simulink model "sldemo_auto_climate_elec"  (Simulink 10.0)
settings: Solver=ode23tb  StartTime=0.0  StopTime=1  RelTol=1e-4  EnableMultiTasking=on
libraries: powerlib x12, simulink x2, simulink_need_slupdate x2
settings Model: FPTRunName=Active  Creator=The MathWorks Inc.  LastModifiedBy=bhisma  ExtModeAutoUpdateStatusClock=off
settings DataIOCC: LimitDataPoints=on  SignalLoggingSaveFormat=ModelDataLogs  SignalLoggingName=sigsOut
settings OptimizationCC: BooleanDataType=off  ExpressionDepthLimit=2147483647  InitFltsAndDblsToZero=on  EfficientMapNaN2IntZero=off
settings DebuggingCC: SaveWithParameterizedLinksMsg=none  SignalResolutionControl=TryResolveAllWithWarning  MultiTaskDSMMsg=warning  MultiTaskCondExecSysMsg=none  FcnCallInpInsideContextMsg=warning  StateNameClashWarn=warning
settings SFSimCC: SimParseCustomCode=off
settings GRTTargetCC: TargetFcnLib=ansi_tfl_tmw.mat  GeneratePreprocessorConditionals=Disable all
settings ConfigComp: CovExternalEMLEnable=off

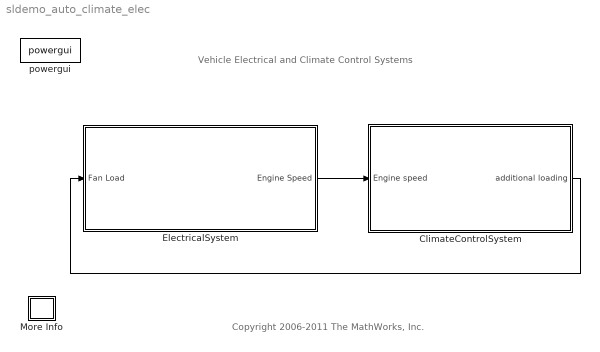
== system sldemo_auto_climate_elec ==
  note: Vehicle Electrical and Climate Control Systems
  note: Copyright 2006-2011 The MathWorks, Inc.
  ClimateControlSystem : Subsystem
  ElectricalSystem : Subsystem
  More Info : Subsystem
      settings: OpenFcn=showdemo(bdroot(gcb))
      mask Display: disp('?')
  powergui : powerlib/powergui  SimulationMode=Continuous  SampleTime=0  frequency=60  Iterations=50  frequencyindice=60  Pbase=100e6  ErrMax=1e-4  UnitsV=kV  UnitsW=MW  buscounter=0  FunctionMessages=off  echomessages=off  EnableUseOfTLC=off  CurrentSourceSwitches=on  DisableSnubberDevices=off  DisableRonSwitches=off  DisableVfSwitches=off  DisplayEquations=off  AutomaticDiscreteSolvers=off  SolverType=Tustin  Interpol=off  ExternalGateDelay=off  methode=off  Ts=0  x0status=blocks  SPID=off  SwTol=0  HookPort=off  NonlinearTolerance=1e-4  nMaxIteration=100  ContinueOnMaxIteration=off  RestoreLinks=no  ResistiveCurrentMeasurement=off  Frange=[0:2:500]  Ylog=off  Xlog=on  ShowGrid=off  save=off  variable=ZData  structure=0  ZoomFFT=on  StartTime=0.0  cycles=1  DisplayStyle=1  fundamental=60  FreqAxis=off  MaxFrequency=1000  frequencyindicesteady=1  RmsSteady=1  display=off
      settings: SourceProductName=Simscape Electrical
  wires:
  ElectricalSystem/1(Engine Speed) -> ClimateControlSystem/1(Engine speed)
  ClimateControlSystem/1(additional loading) -> ElectricalSystem/1(Fan Load)

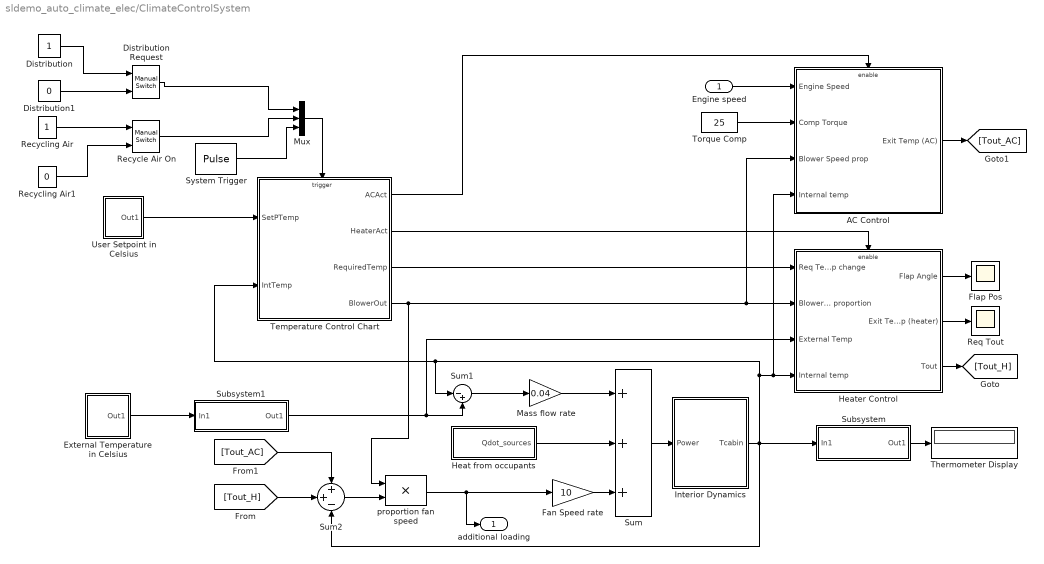
== system sldemo_auto_climate_elec/ClimateControlSystem ==
  Engine speed : Inport
  AC Control : Subsystem  TreatAsAtomicUnit=on
  "Distribution " : Constant
  Distribution Request : simulink/Signal Routing/Manual Switch  sw=0  action=0  varsize=off
      settings: SourceProductName=Simulink  SourceProductBaseCode=SL
  "Distribution1 " : Constant  Value=0
  External Temperature in Celsius : Subsystem  mask(variable){x=18}
      mask prompts: x "Enter the external temperature"
      mask init:
      | set_param('sldemo_auto_climate_elec/ClimateControlSystem/External Temperature in Celsius/External Temp','Value',num2str(x))
      mask Display: disp(x);
  Fan Speed rate : Gain  Gain=10  SaturateOnIntegerOverflow=on  OutDataTypeStr=Inherit: Same as input  ParamDataTypeStr=Inherit: Same as input
  Flap Pos : Scope
  Heat from occupants : Subsystem  mask(Heat from occupants){N=1}
      mask prompts: N "Number of occupants:"
      settings: AttributesFormatString=No. of occupants: %<N>
      mask Display: disp('Heat Sources')
  Heater Control : Subsystem  TreatAsAtomicUnit=on
  Interior Dynamics : Subsystem  mask(Vehicle Cabin Dynamics){}
      mask Display: image(imread([matlabroot,'/toolbox/simulink/simdemos/automotive/html/car_int.jpg']))
  Mass flow rate : Gain  Gain=0.04  SaturateOnIntegerOverflow=on  OutDataTypeStr=Inherit: Same as input  ParamDataTypeStr=Inherit: Same as input
  Mux : Mux  Inputs=3
  Recycle Air On : simulink/Signal Routing/Manual Switch  sw=0  action=0  varsize=off
      settings: SourceProductName=Simulink  SourceProductBaseCode=SL
  Recycling Air : Constant
  Recycling Air1 : Constant  Value=0
  Req Tout : Scope
  Subsystem : Subsystem
      mask Display: disp('Kelvin to Celsius')
  Subsystem1 : Subsystem
      mask Display: disp('Celsius to Kelvin')
  Sum : Sum  Inputs=+++  SaturateOnIntegerOverflow=on  InputSameDT=on  OutDataTypeStr=Inherit: Same as first input
  Sum1 : Sum  Inputs=|-+  SaturateOnIntegerOverflow=on  InputSameDT=on  OutDataTypeStr=Inherit: Same as first input
  Sum2 : Sum  Inputs=++-  SaturateOnIntegerOverflow=on  InputSameDT=on  OutDataTypeStr=Inherit: Same as first input
  System Trigger : DiscretePulseGenerator  PulseType=Time based  Period=1/60  PulseWidth=50
  Temperature Control Chart : Stateflow chart  TreatAsAtomicUnit=on
  Thermometer Display : Display
  Torque Comp : Constant  Value=25
  User Setpoint in Celsius : Subsystem  mask{USet=9}
      mask prompts: USet "Enter the Temperature you require"
      mask init:
      | set_param('sldemo_auto_climate_elec/ClimateControlSystem/User Setpoint in Celsius/User Setpoint','Value',num2str(USet))
      mask Display: disp(num2str(USet))
  proportion fan speed : Product  SaturateOnIntegerOverflow=on  InputSameDT=on  OutDataTypeStr=Inherit: Same as first input
  additional loading : Outport
  wires:
  Distribution Request/1 -> Mux/1
  "Distribution "/1 -> Distribution Request/1
  "Distribution1 "/1 -> Distribution Request/2
  Recycling Air1/1 -> Recycle Air On/2
  User Setpoint in Celsius/1(Out1) -> Temperature Control Chart/1(SetPTemp)
  Recycling Air/1 -> Recycle Air On/1
  Recycle Air On/1 -> Mux/2
  System Trigger/1 -> Mux/3
  Interior Dynamics/1("Tcabin ") -> AC Control/4(Internal temp), Heater Control/4(Internal temp), Temperature Control Chart/2(IntTemp), Sum1/1, Sum2/3, Subsystem/1(In1)
  Subsystem/1(Out1) -> Thermometer Display/1
  Heat from occupants/1(Qdot_sources) -> Sum/2
  External Temperature in Celsius/1(Out1) -> Subsystem1/1(In1)
  Mass flow rate/1 -> Sum/1
  Sum1/1 -> Mass flow rate/1
  Subsystem1/1(Out1) -> Heater Control/3(External Temp), Sum1/2
  Fan Speed rate/1 -> Sum/3
  Sum2/1 -> proportion fan speed/2
  Temperature Control Chart/4(BlowerOut) -> AC Control/3(Blower Speed prop), Heater Control/2(Blower Speed proportion), proportion fan speed/1
  proportion fan speed/1 -> additional loading/1, Fan Speed rate/1
  Temperature Control Chart/2(" HeaterAct") -> Heater Control/Enable
  Heater Control/1(Flap Angle) -> Flap Pos/1
  Heater Control/2(Exit Temp (heater)) -> Req Tout/1
  Heater Control/3(Tout) -> [Tout_H]
  [Tout_H] -> Sum2/2
  Temperature Control Chart/1(" ACAct") -> AC Control/Enable
  [Tout_AC] -> Sum2/1
  Torque Comp/1 -> AC Control/2(Comp Torque)
  Temperature Control Chart/3(RequiredTemp) -> Heater Control/1(Req Temp change)
  AC Control/1(Exit Temp (AC)) -> [Tout_AC]
  Engine speed/1 -> AC Control/1(Engine Speed)
  Mux/1 -> Temperature Control Chart/Trigger
  Sum/1 -> Interior Dynamics/1(Power)

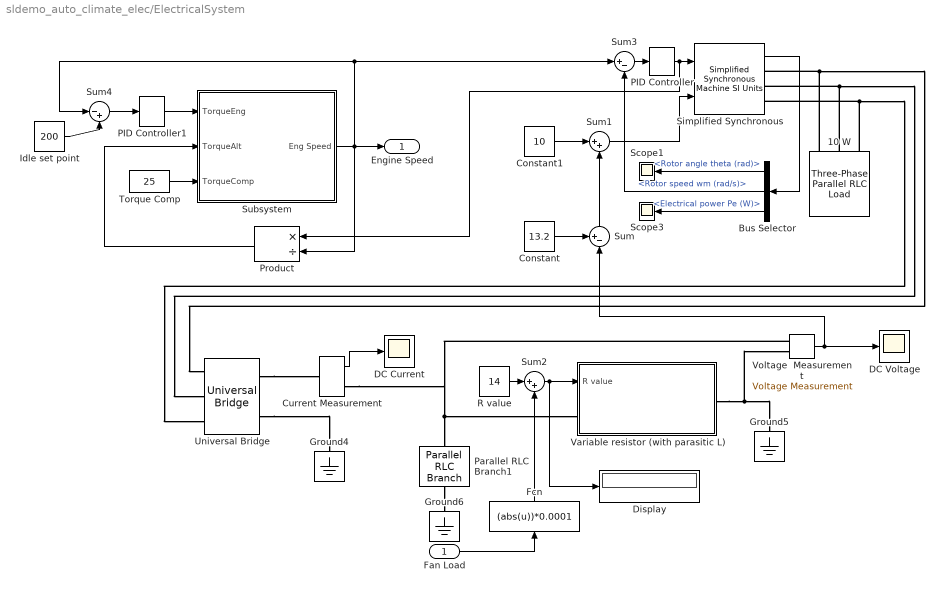
== system sldemo_auto_climate_elec/ElectricalSystem ==
  Fan Load : Inport
  " DC Current" : Scope
  10 W : powerlib/Elements/Three-Phase Parallel RLC Load  LConnTagsString=A|B|C  Configuration=Y (grounded)  NominalVoltage=20  NominalFrequency=60  ActivePower=1  InductivePower=0  CapacitivePower=0  Measurements=None  LoadType=constant Z
      settings: SourceProductName=Simscape Electrical
  Bus Selector : BusSelector  OutputSignals=Rotor angle theta (rad),Rotor speed wm (rad/s),Electrical power Pe (W)
  Constant : Constant  Value=13.2
  Constant1 : Constant  Value=10
  Current Measurement : powerlib/Measurements/Current Measurement  PhasorSimulation=off  OutputType=Magnitude  PSBequivalent=0
      settings: SourceProductName=Simscape Electrical
  DC Voltage : Scope
  Display : Display
  Fcn : Fcn  Expr=(abs(u))*0.0001
  Ground4 : powerlib/Elements/Ground  LConnTagsString=a
      settings: SourceProductName=Simscape Electrical
  Ground5 : powerlib/Elements/Ground  LConnTagsString=a
      settings: SourceProductName=Simscape Electrical
  Ground6 : powerlib/Elements/Ground  LConnTagsString=a
      settings: SourceProductName=Simscape Electrical
  Idle set point : Constant  Value=200
  PID Controller : simulink_need_slupdate/PID Controller  P=2  I=8  D=1
      settings: SourceProductName=Simulink
  PID Controller1 : simulink_need_slupdate/PID Controller  P=2  I=8  D=0
      settings: SourceProductName=Simulink
  Parallel RLC Branch1 : powerlib/Elements/Parallel RLC Branch  LConnTagsString=a  RConnTagsString=__new0  BranchType=RC  Resistance=100  Inductance=1.0  SetiL0=off  InitialCurrent=0  Capacitance=50e-06  Setx0=off  InitialVoltage=0  Measurements=None
      settings: SourceProductName=Simscape Electrical
  Product : Product  Inputs=*/  SaturateOnIntegerOverflow=on  InputSameDT=on  OutDataTypeStr=Inherit: Same as first input
  R value : Constant  Value=14
  Scope1 : Scope
  Scope3 : Scope
  "Simplified Synchronous " : powerlib/Machines/Simplified Synchronous Machine SI Units  ConnectionType=3-wire Y  MechanicalLoad=Mechanical power Pm  NominalParameters=[ 750, 20, 60 ]  Mechanical=[ inf, 0, 3]  InternalRL=[ 0.1, 2.15e-5 ]  InitialConditions="[ 0   0   0,0,0   0,0,0 ]"  Units=1  LoadFlowParameters=[1,0,0,0,0]  TsPowergui=0  TsBlock=-1  BusType=PV  Pref=0  Qref=0  Qmin=-inf  Qmax=+inf  PLF=0  QLF=0
      settings: SourceProductName=Simscape Electrical  SourceProductBaseCode=PS
  Subsystem : Subsystem
  Sum : Sum  Inputs=+-|  SaturateOnIntegerOverflow=on  InputSameDT=on  OutDataTypeStr=Inherit: Same as first input
  Sum1 : Sum  Inputs=|++  SaturateOnIntegerOverflow=on  InputSameDT=on  OutDataTypeStr=Inherit: Same as first input
  Sum2 : Sum  Inputs=|++  SaturateOnIntegerOverflow=on  InputSameDT=on  OutDataTypeStr=Inherit: Same as first input
  Sum3 : Sum  Inputs=|+-  SaturateOnIntegerOverflow=on  InputSameDT=on  OutDataTypeStr=Inherit: Same as first input
  Sum4 : Sum  Inputs=|-+  SaturateOnIntegerOverflow=on  InputSameDT=on  OutDataTypeStr=Inherit: Same as first input
  Torque Comp : Constant  Value=25
  Universal Bridge : powerlib/Power Electronics/Universal Bridge  Arms=3  SnubberResistance=1e10  SnubberCapacitance=100e-09  Device=Diodes  Ron=0.01  Lon=0  ForwardVoltages="[  0  0  ]"  ForwardVoltage=0.8  GTOparameters=[ 10e-6 , 20e-6 ]  IGBTparameters=[ 1e-6 , 2e-6 ]  Measurements=None  Measurements_2=None  converterType=Rectifier
      settings: SourceProductName=Simscape Electrical
  "Variable resistor (with parasitic L) " : Subsystem
      mask Display: disp('Variable Resistor');
  Voltage  Measurement : powerlib/Measurements/Voltage Measurement  PhasorSimulation=off  OutputType=Magnitude  PSBequivalent=0
      settings: SourceProductName=Simscape Electrical
  Engine Speed : Outport  InitialOutput=0
  wires:
  Constant1/1 -> Sum1/1
  Sum/1 -> Sum1/2
  Sum2/1 -> Display/1, "Variable resistor (with parasitic L) "/1(R value)
  R value/1 -> Sum2/1
  Fan Load/1 -> Fcn/1
  Subsystem/1(Eng Speed) -> Sum3/1, Sum4/1, Product/2, Engine Speed/1
  Torque Comp/1 -> Subsystem/3(TorqueComp)
  Constant/1 -> Sum/1
  Sum3/1 -> PID Controller/1
  Sum4/1 -> PID Controller1/1
  Idle set point/1 -> Sum4/2
  PID Controller1/1 -> Subsystem/1(TorqueEng)
  Product/1 -> Subsystem/2(TorqueAlt)
  Fcn/1 -> Sum2/2
  Sum1/1 -> "Simplified Synchronous "/2
  Voltage  Measurement/1 -> DC Voltage/1, Sum/2
  Current Measurement/1 -> " DC Current"/1
  "Simplified Synchronous "/1 -> Bus Selector/1
  Bus Selector/1 -> Scope1/1  "<Rotor angle theta (rad)>"
  Bus Selector/3 -> Scope3/1  "<Electrical power Pe (W)>"
  PID Controller/1 -> "Simplified Synchronous "/1, Product/1
  Bus Selector/2 -> Sum3/2  "<Rotor speed wm (rad/s)>"
  connections:
  10 W/LConn2 -- Universal Bridge/LConn2 -- "Simplified Synchronous "/RConn2
  10 W/LConn1 -- Universal Bridge/LConn1 -- "Simplified Synchronous "/RConn1
  10 W/LConn3 -- Universal Bridge/LConn3 -- "Simplified Synchronous "/RConn3
  Universal Bridge/RConn2 -- Ground4/LConn1
  Parallel RLC Branch1/RConn1 -- Ground6/LConn1
  Universal Bridge/RConn1 -- Current Measurement/LConn1
  Current Measurement/RConn1 -- Voltage  Measurement/LConn1 -- Parallel RLC Branch1/LConn1 -- "Variable resistor (with parasitic L) "/LConn1
  "Variable resistor (with parasitic L) "/RConn1 -- Ground5/LConn1 -- Voltage  Measurement/LConn2

== system sldemo_auto_climate_elec/More Info ==

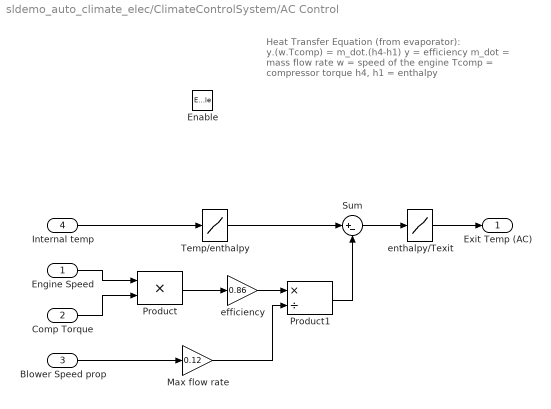
== system sldemo_auto_climate_elec/ClimateControlSystem/AC Control ==
  note: Heat Transfer Equation (from evaporator):
      |
      | y.(w.Tcomp) = m_dot.(h4-h1)
      |
      | y = efficiency
      | m_dot = mass flow rate
      | w = speed of the engine
      | Tcomp = compressor torque
      | h4, h1 = enthalpy
  Engine Speed : Inport
  Comp Torque : Inport  Port=2
  Blower Speed prop : Inport  Port=3
  Internal temp : Inport  Port=4
  Enable : EnablePort  StatesWhenEnabling=reset  PropagateVarSize=During execution  ZeroCross=off
  Max flow rate : Gain  Gain=0.12  SaturateOnIntegerOverflow=on  OutDataTypeStr=Inherit: Same as input  ParamDataTypeStr=Inherit: Same as input
  Product : Product  SaturateOnIntegerOverflow=on  InputSameDT=on  OutDataTypeStr=Inherit: Same as first input
  Product1 : Product  Inputs=*/  SaturateOnIntegerOverflow=on  InputSameDT=on  OutDataTypeStr=Inherit: Same as first input
  Sum : Sum  Inputs=|+-  SaturateOnIntegerOverflow=on  InputSameDT=on  OutDataTypeStr=Inherit: Same as first input
  Temp/enthalpy : Lookup_n-D  NumberOfTableDimensions=1  BreakpointsForDimension1=[220 230 240 250 260 270 280 285 290 295 300 305 310 315 320]  Table=[219.97 230.02 240.02 250.05 260.09 270.11 280.13 285.14 290.16 295.17 300.19 305.22 310.24 315.27 320.29]  SaturateOnIntegerOverflow=on  InputSameDT=on
  efficiency : Gain  Gain=0.86  SaturateOnIntegerOverflow=on  OutDataTypeStr=Inherit: Same as input  ParamDataTypeStr=Inherit: Same as input
  enthalpy/Texit : Lookup_n-D  NumberOfTableDimensions=1  BreakpointsForDimension1=[219.97 230.02 240.02 250.05 260.09 270.11 280.13 285.14 290.16 295.17 300.19 305.22 310.24 315.27 320.29]  Table=[220 230 240 250 260 270 280 285 290 295 300 305 310 315 320]  SaturateOnIntegerOverflow=on  InputSameDT=on
  Exit Temp (AC) : Outport  OutputWhenDisabled=reset  InitialOutput=0
  wires:
  Sum/1 -> enthalpy/Texit/1
  Product1/1 -> Sum/2
  Temp/enthalpy/1 -> Sum/1
  Internal temp/1 -> Temp/enthalpy/1
  enthalpy/Texit/1 -> Exit Temp (AC)/1
  Max flow rate/1 -> Product1/2
  Blower Speed prop/1 -> Max flow rate/1
  efficiency/1 -> Product1/1
  Product/1 -> efficiency/1
  Comp Torque/1 -> Product/2
  Engine Speed/1 -> Product/1

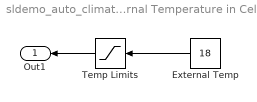
== system sldemo_auto_climate_elec/ClimateControlSystem/External Temperature in Celsius ==
  External Temp : Constant  Value=18
  Temp Limits : Saturate  UpperLimit=100  LowerLimit=-99
  Out1 : Outport
  wires:
  Temp Limits/1 -> Out1/1
  External Temp/1 -> Temp Limits/1

== system sldemo_auto_climate_elec/ClimateControlSystem/Heat from occupants ==
  No of occupants : Gain  Gain=N  SaturateOnIntegerOverflow=on  OutDataTypeStr=Inherit: Same as input  ParamDataTypeStr=Inherit: Same as input
  Power per occupant [W] : Constant  Value=100
  Qdot_sources : Outport
  wires:
  Power per occupant [W]/1 -> No of occupants/1
  No of occupants/1 -> Qdot_sources/1  "Qdot_sources"

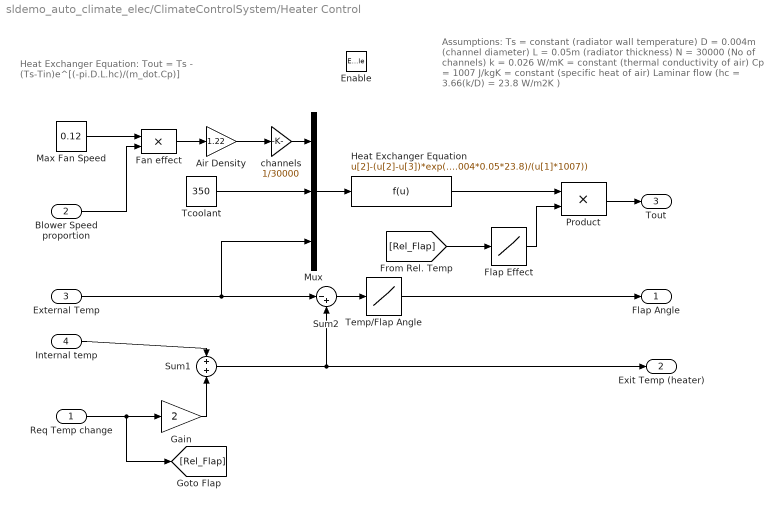
== system sldemo_auto_climate_elec/ClimateControlSystem/Heater Control ==
  note: Assumptions:
      | Ts = constant (radiator wall temperature)
      | D = 0.004m (channel diameter)
      | L = 0.05m (radiator thickness)
      | N = 30000 (No of channels)
      |
      | k = 0.026 W/mK = constant (thermal conductivity of air)
      | Cp = 1007 J/kgK = constant (specific heat of air)
      | Laminar flow (hc = 3.66(k/D) = 23.8 W/m2K )
  note: Heat Exchanger Equation:
      | Tout = Ts - (Ts-Tin)e^[(-pi.D.L.hc)/(m_dot.Cp)]
  Req Temp change : Inport
  Blower Speed proportion : Inport  Port=2
  External Temp : Inport  Port=3
  Internal temp : Inport  Port=4
  Enable : EnablePort  StatesWhenEnabling=reset  PropagateVarSize=During execution  ZeroCross=off
  Air Density : Gain  Gain=1.22  SaturateOnIntegerOverflow=on  OutDataTypeStr=Inherit: Same as input  ParamDataTypeStr=Inherit: Same as input
  Fan effect : Product  SaturateOnIntegerOverflow=on  InputSameDT=on  OutDataTypeStr=Inherit: Same as first input
  Flap Effect : Lookup_n-D  NumberOfTableDimensions=1  BreakpointsForDimension1="[0 3 5 10 50  90 100 200 ]"  Table="[0 300 100  10 10  10 3 1]"  SaturateOnIntegerOverflow=on  InputSameDT=on
  Gain : Gain  Gain=2  SaturateOnIntegerOverflow=on  OutDataTypeStr=Inherit: Same as input  ParamDataTypeStr=Inherit: Same as input
  Heat Exchanger Equation : Fcn  Expr=u[2]-(u[2]-u[3])*exp(-(pi*0.004*0.05*23.8)/(u[1]*1007))
  Max Fan Speed : Constant  Value=0.12
  Mux : Mux  Inputs=3
  Product : Product  SaturateOnIntegerOverflow=on  InputSameDT=on  OutDataTypeStr=Inherit: Same as first input
  Sum1 : Sum  SaturateOnIntegerOverflow=on  InputSameDT=on  OutDataTypeStr=Inherit: Same as first input
  Sum2 : Sum  Inputs=|-+  SaturateOnIntegerOverflow=on  InputSameDT=on  OutDataTypeStr=Inherit: Same as first input
  "Tcoolant " : Constant  Value=350
  Temp/Flap Angle : Lookup_n-D  NumberOfTableDimensions=1  BreakpointsForDimension1=[0 10 20 30 40 50 60 75 100 200]  Table=[0 20 30 45 60 75 90 90 90 90]  SaturateOnIntegerOverflow=on  InputSameDT=on
  channels : Gain  Gain=1/30000  SaturateOnIntegerOverflow=on  OutDataTypeStr=Inherit: Same as input  ParamDataTypeStr=Inherit: Same as input
  Flap Angle : Outport  OutputWhenDisabled=reset  InitialOutput=0
  Exit Temp (heater) : Outport  Port=2  OutputWhenDisabled=reset  InitialOutput=0
  Tout : Outport  Port=3  OutputWhenDisabled=reset  InitialOutput=0
  wires:
  Heat Exchanger Equation/1 -> Product/1
  External Temp/1 -> Mux/3, Sum2/1
  Blower Speed proportion/1 -> Fan effect/2
  Max Fan Speed/1 -> Fan effect/1
  Fan effect/1 -> Air Density/1
  Mux/1 -> Heat Exchanger Equation/1
  Air Density/1 -> channels/1
  channels/1 -> Mux/1
  "Tcoolant "/1 -> Mux/2
  Product/1 -> Tout/1
  Temp/Flap Angle/1 -> Flap Angle/1
  Sum2/1 -> Temp/Flap Angle/1
  Internal temp/1 -> Sum1/1
  Gain/1 -> Sum1/2
  Sum1/1 -> Exit Temp (heater)/1, Sum2/2
  Req Temp change/1 -> Gain/1, [Rel_Flap]
  Flap Effect/1 -> Product/2
  [Rel_Flap] -> Flap Effect/1

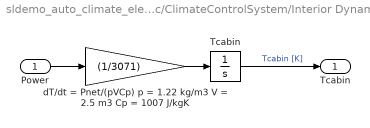
== system sldemo_auto_climate_elec/ClimateControlSystem/Interior Dynamics ==
  Power : Inport
  Tcabin : Integrator  InitialCondition=291  ZeroCross=off
  dT/dt = Pnet/(pVCp) p = 1.22 kg/m3 V = 2.5 m3 Cp = 1007 J/kgK : Gain  Gain=(1/3071)  SaturateOnIntegerOverflow=on  OutDataTypeStr=Inherit: Same as input  ParamDataTypeStr=Inherit: Same as input
  "Tcabin " : Outport
  wires:
  dT/dt = Pnet/(pVCp) p = 1.22 kg/m3 V = 2.5 m3 Cp = 1007 J/kgK/1 -> Tcabin/1
  Power/1 -> dT/dt = Pnet/(pVCp) p = 1.22 kg/m3 V = 2.5 m3 Cp = 1007 J/kgK/1
  Tcabin/1 -> "Tcabin "/1  "Tcabin [K]"

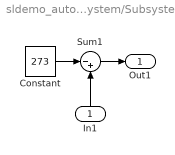
== system sldemo_auto_climate_elec/ClimateControlSystem/Subsystem ==
  In1 : Inport
  Constant : Constant  Value=273
  Sum1 : Sum  Inputs=|-+  SaturateOnIntegerOverflow=on  InputSameDT=on  OutDataTypeStr=Inherit: Same as first input
  Out1 : Outport
  wires:
  Sum1/1 -> Out1/1
  In1/1 -> Sum1/2
  Constant/1 -> Sum1/1

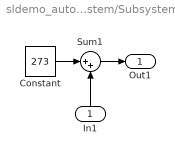
== system sldemo_auto_climate_elec/ClimateControlSystem/Subsystem1 ==
  In1 : Inport
  Constant : Constant  Value=273
  Sum1 : Sum  Inputs=|++  SaturateOnIntegerOverflow=on  InputSameDT=on  OutDataTypeStr=Inherit: Same as first input
  Out1 : Outport
  wires:
  Constant/1 -> Sum1/1
  In1/1 -> Sum1/2
  Sum1/1 -> Out1/1

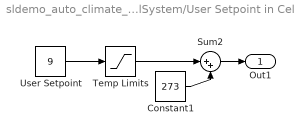
== system sldemo_auto_climate_elec/ClimateControlSystem/User Setpoint in Celsius ==
  Constant1 : Constant  Value=273
  Sum2 : Sum  Inputs=|++  SaturateOnIntegerOverflow=on  InputSameDT=on  OutDataTypeStr=Inherit: Same as first input
  Temp Limits : Saturate  UpperLimit=100  LowerLimit=-99
  User Setpoint : Constant  Value=9
  Out1 : Outport
  wires:
  Sum2/1 -> Out1/1
  User Setpoint/1 -> Temp Limits/1
  Constant1/1 -> Sum2/2
  Temp Limits/1 -> Sum2/1

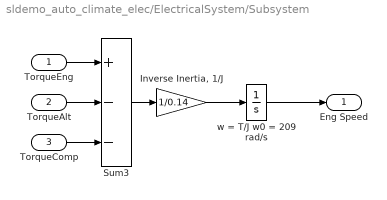
== system sldemo_auto_climate_elec/ElectricalSystem/Subsystem ==
  TorqueEng : Inport
  TorqueAlt : Inport  Port=2
  TorqueComp : Inport  Port=3
  "Inverse Inertia, 1/J" : Gain  Gain=1/0.14  SaturateOnIntegerOverflow=on  OutDataTypeStr=Inherit: Same as input  ParamDataTypeStr=Inherit: Same as input
  Sum3 : Sum  Inputs=+--  SaturateOnIntegerOverflow=on  InputSameDT=on  OutDataTypeStr=Inherit: Same as first input
  w = T/J w0 = 209 rad/s : Integrator  InitialCondition=209.48  ZeroCross=off
  Eng Speed : Outport  InitialOutput=0
  wires:
  "Inverse Inertia, 1/J"/1 -> w = T/J w0 = 209 rad/s/1
  w = T/J w0 = 209 rad/s/1 -> Eng Speed/1
  Sum3/1 -> "Inverse Inertia, 1/J"/1
  TorqueEng/1 -> Sum3/1
  TorqueAlt/1 -> Sum3/2
  TorqueComp/1 -> Sum3/3

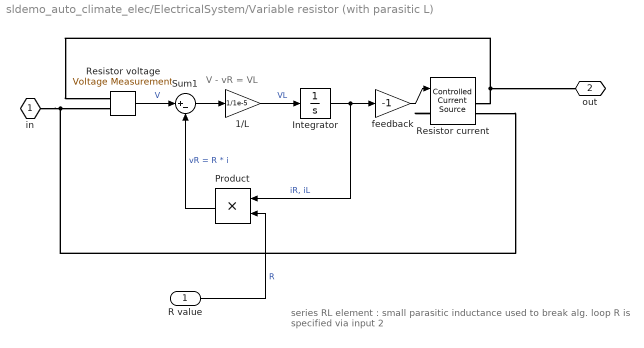
== system sldemo_auto_climate_elec/ElectricalSystem/Variable resistor (with parasitic L)  ==
  note: V - vR = VL
  note: series RL element : small parasitic inductance used to break alg. loop
      | R is specified via input 2
  R value : Inport
  1/L : Gain  Gain=1/1e-5  SaturateOnIntegerOverflow=on  OutDataTypeStr=Inherit: Same as input  ParamDataTypeStr=Inherit: Same as input
  Integrator : Integrator  ZeroCross=off
  Product : Product  SaturateOnIntegerOverflow=on  InputSameDT=on  OutDataTypeStr=Inherit: Same as first input
  Resistor current : powerlib/Electrical Sources/Controlled Current Source  Initialize=on  Source_Type=AC  Amplitude=0  Phase=0  Frequency=0  Measurements=None
      settings: SourceProductName=Simscape Electrical
  Resistor voltage : powerlib/Measurements/Voltage Measurement  PhasorSimulation=off  OutputType=Magnitude  PSBequivalent=0
      settings: SourceProductName=Simscape Electrical
  Sum1 : Sum  Inputs=|+-  SaturateOnIntegerOverflow=on  InputSameDT=on  OutDataTypeStr=Inherit: Same as first input
  feedback : Gain  Gain=-1  SaturateOnIntegerOverflow=on  OutDataTypeStr=Inherit: Same as input  ParamDataTypeStr=Inherit: Same as input
  in : PMIOPort  Side=Left
  out : PMIOPort  Port=2  Side=Right
  wires:
  Sum1/1 -> 1/L/1
  Integrator/1 -> Product/1, feedback/1  "iR, iL"
  1/L/1 -> Integrator/1  "VL"
  R value/1 -> Product/2  "R"
  Product/1 -> Sum1/2  "vR = R * i"
  Resistor voltage/1 -> Sum1/1  "V"
  feedback/1 -> Resistor current/1
  connections:
  Resistor current/RConn1 -- out/RConn1 -- Resistor voltage/LConn1
  in/RConn1 -- Resistor voltage/LConn2 -- Resistor current/LConn1

== stateflow chart ClimateControlSystem/Temperature Control Chart ==
  state Blower [parallel]
    during:setpoint_calc();
    settings: executionOrder=1
    state Blower_off
      entry:BlowerOut=0.0;
    state Blower_on
      state Blower_1
        entry:BlowerOut=0.2;
      state Blower_2
        entry:BlowerOut=0.4;
      state Blower_3
        entry:BlowerOut=0.6;
      state Blower_4
        entry:BlowerOut=0.8;
      state Blower_5
        entry:BlowerOut=1.0;
      (default) -> Blower_1
      Blower_on -> Blower_1 [order 5] : E[!in(Blower_1) && in_temp_range(1.5,5)]
      Blower_on -> Blower_2 [order 4] : E[!in(Blower_2) && in_temp_range(7,10)]
      Blower_on -> Blower_3 [order 3] : E[!in(Blower_3) && in_temp_range(12,15)]
      Blower_on -> Blower_4 [order 2] : E[!in(Blower_4) && in_temp_range(17,20)]
      Blower_on -> Blower_5 [order 1] : E[!in(Blower_5) && in_temp_range(22,200)]
    state setpoint_calc() [function]
      (default) -> (junction 33) : {RequiredTemp = SetPTemp-IntTemp;}
      (junction 33) -> (junction 34) [order 1] : [RequiredTemp<0.0]
          | {absTempDiff = -RequiredTemp;}
      (junction 33) -> (junction 35) [order 2] : {absTempDiff = RequiredTemp;}
    state b = in_temp_range(minTemp,maxTemp) [function]
      (default) -> (junction 42) : {b = (absTempDiff>minTemp) &&  ...
          |         (absTempDiff<maxTemp);}
    (default) -> Blower_off
    Blower_off -> Blower_on : E[in_temp_range(.5,203)]
    Blower_on -> Blower_off [order 1] : E[absTempDiff>203 || absTempDiff<=0.5]
  state Heater_AC [parallel]
    settings: executionOrder=2
    state H_offAC_off
    state ACAct
    state HeaterAct
    ACAct -> H_offAC_off : E[SetPTemp-IntTemp>=-0.5]
    HeaterAct -> H_offAC_off : E[SetPTemp-IntTemp<=0.5]
    H_offAC_off -> HeaterAct [order 2] : E[SetPTemp-IntTemp>0.5]
    H_offAC_off -> ACAct [order 1] : E[SetPTemp-IntTemp<-0.5]
    (default) -> H_offAC_off
  state AirDist [parallel]
    settings: executionOrder=3
    state Feet
    state Face
    state Defrost
    (default) -> Face
    Feet -> Defrost : DistReq
    Face -> Feet : DistReq
    Defrost -> Face : DistReq
  state Recyc_Air [parallel]
    settings: executionOrder=4
    state Recyc_on
    state Recyc_off
    (default) -> Recyc_on
    Recyc_on -> Recyc_off [order 2] : RecycReq
    Recyc_off -> Recyc_on : RecycReq
    Recyc_on -> Recyc_off [order 1] : en(AirDist.Defrost)
  data: minTemp function_input double; b function_output boolean; maxTemp function_input double; ACAct output unknown; SetPTemp input double; IntTemp input double; HeaterAct output unknown; RequiredTemp output double; BlowerOut output double; absTempDiff local double
  events: DistReq input EITHER_EDGE_EVENT; RecycReq input EITHER_EDGE_EVENT; E input EITHER_EDGE_EVENT
